simulink model "rotary_mass_spring_damp"  (R2020a)
settings: Solver=VariableStepAuto  StartTime=0.0  StopTime=50  RelTol=1e-3
model workspace (MAT data in the model file):
  B = 5
  C = 1
  J = Simulink.Parameter
  J.Value = 10
  J.Description = 'Inertia'
  J.DataType = 'auto'
  J.Dimensions = [1 1]
  K = 5
undefined symbols (not defined in the file): NULL, serial
libraries: instrumentlib x3
settings Model: Creator=Jordan  LastModifiedBy=Jordan

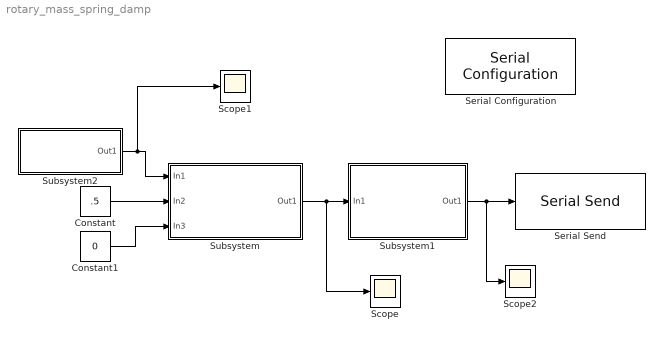
== system rotary_mass_spring_damp ==
  Constant : Constant  Value=.5
  Constant1 : Constant  Value=0
  Scope : Scope
  Scope1 : Scope
  Scope2 : Scope
  Serial Configuration : instrumentlib/Serial Configuration  Priority=-200000  ComPortMenu=COM3  ComPort=COM3  ObjConstructor=serial('COM3');  BaudRate=115200  DataBits=8  Parity=none  StopBits=1  FlowControl=none  Timeout=.1  ByteOrder=LittleEndian
  Serial Send : instrumentlib/Serial Send  ComPortMenu=COM3  ComPort=COM3  ObjConstructor=serial('COM3');  Terminator=NULL ('\0')  EnableBlockingMode=on
  Subsystem : Subsystem
  Subsystem1 : Subsystem
  Subsystem2 : Subsystem
  wires:
  Subsystem1/1(Out1) -> Scope2/1, Serial Send/1
  Subsystem/1(Out1) -> Scope/1, Subsystem1/1(In1)
  Subsystem2/1(Out1) -> Scope1/1, Subsystem/1(In1)
  Constant/1 -> Subsystem/2(In2)
  Constant1/1 -> Subsystem/3(In3)

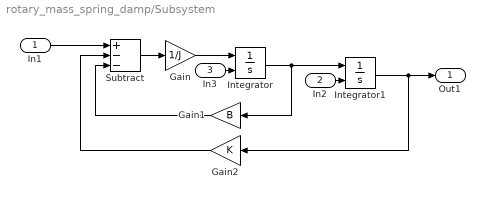
== system rotary_mass_spring_damp/Subsystem ==
  In1 : Inport
  In2 : Inport  Port=2
  In3 : Inport  Port=3
  Gain : Gain  Gain=1/J
  Gain1 : Gain  Gain=B
  Gain2 : Gain  Gain=K
  Integrator : Integrator  InitialConditionSource=external
  Integrator1 : Integrator  InitialConditionSource=external
  Subtract : Sum  Inputs=+--
  Out1 : Outport
  wires:
  In1/1 -> Subtract/1
  Gain2/1 -> Subtract/2
  Gain1/1 -> Subtract/3
  Integrator1/1 -> Out1/1, Gain2/1
  In2/1 -> Integrator1/2
  Subtract/1 -> Gain/1
  Gain/1 -> Integrator/1
  Integrator/1 -> Gain1/1, Integrator1/1
  In3/1 -> Integrator/2

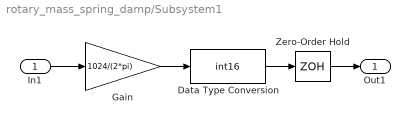
== system rotary_mass_spring_damp/Subsystem1 ==
  In1 : Inport
  Data Type Conversion : DataTypeConversion  OutDataTypeStr=int16
  Gain : Gain  Gain=1024/(2*pi)
  Zero-Order Hold : ZeroOrderHold  SampleTime=-1
  Out1 : Outport
  wires:
  In1/1 -> Gain/1
  Gain/1 -> Data Type Conversion/1
  Zero-Order Hold/1 -> Out1/1
  Data Type Conversion/1 -> Zero-Order Hold/1

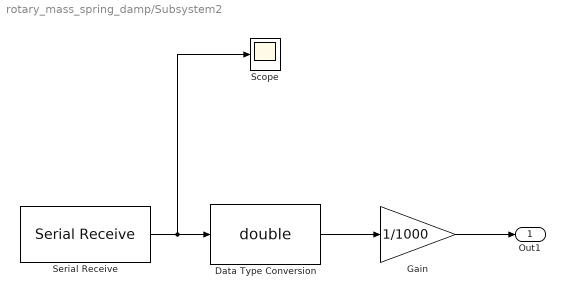
== system rotary_mass_spring_damp/Subsystem2 ==
  Data Type Conversion : DataTypeConversion  OutDataTypeStr=double
  Gain : Gain  Gain=1/1000
  Scope : Scope
  Serial Receive : instrumentlib/Serial Receive  ComPortMenu=COM3  ComPort=COM3  ObjConstructor=serial('COM3');  Terminator=NULL ('\0')  DataSize="[1  1]"  DataType=int16  EnableBlockingMode=on  ActionDataUnavailable=Output last received value  CustomValue=0  SampleTime=.1
  Out1 : Outport
  wires:
  Gain/1 -> Out1/1
  Data Type Conversion/1 -> Gain/1
  Serial Receive/1 -> Scope/1, Data Type Conversion/1
